simulink model "DinamicaActuadorTesis"  (R2021b)
settings: Solver=VariableStepAuto  StartTime=0.0  StopTime=5  RelTol=1e-3
libraries: slpidlib x4
(part 1 of 2)
settings Model: Creator=fabia  LastModifiedBy=fabia

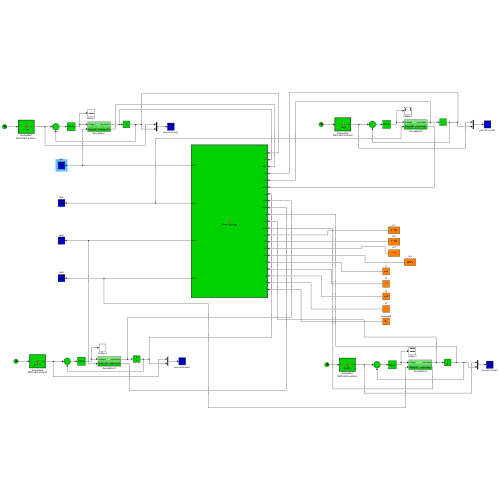
[thumbnail: Simulink's stored preview of the top-level diagram]
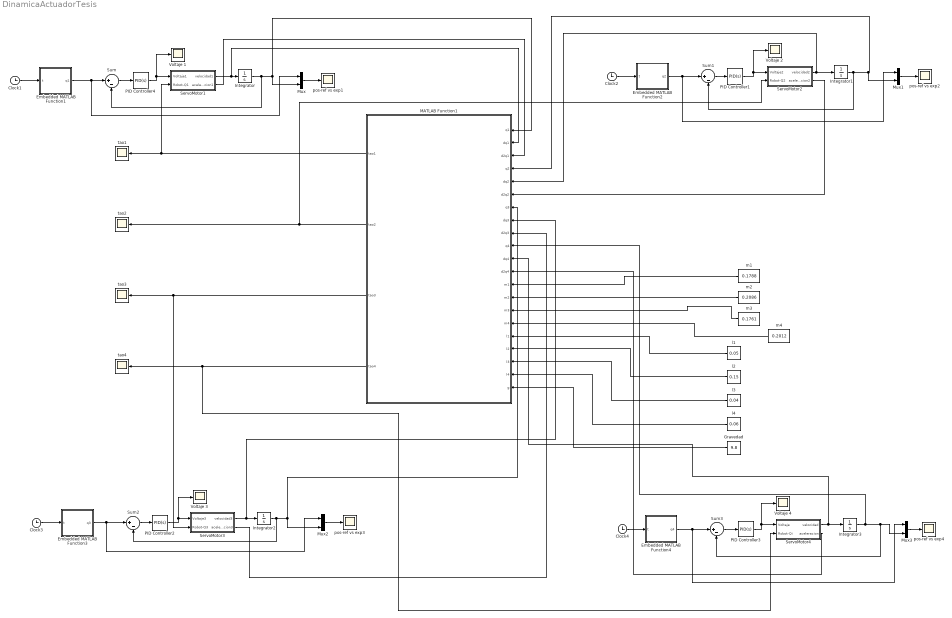
== system DinamicaActuadorTesis ==
  Clock{1..4} (4 alike) : Clock
      settings: Decimation=1000
  Embedded MATLAB Function1 : MATLAB Function  TreatAsAtomicUnit=on
  Embedded MATLAB Function2 : MATLAB Function  TreatAsAtomicUnit=on
  Embedded MATLAB Function3 : MATLAB Function  TreatAsAtomicUnit=on
  Embedded MATLAB Function4 : MATLAB Function  TreatAsAtomicUnit=on
  Gravedad : Constant  Value=9.8
  Integrator{,1..3} (4 alike) : Integrator
  MATLAB Function1 : MATLAB Function  TreatAsAtomicUnit=on
  Mux{,1..3} (4 alike) : Mux  Inputs=2
  PID Controller1 : slpidlib/PID Controller  Controller=PID  Form=Parallel  TimeDomain=Continuous-time  UseExternalTs=off  SampleTime=-1  IntegratorMethod=Forward Euler  FilterMethod=Forward Euler  ControllerParametersSource=internal  P=21468.8085757443  I=3151896.46029539  D=35.5661379721855  UseFilter=on  N=28467.1470128127  TunerSelectOption=Transfer Function Based (PID Tuner App)  InitialConditionSource=internal  InitialConditionForIntegrator=0  InitialConditionForFilter=0  DifferentiatorICPrevScaledInput=0  ExternalReset=none  TrackingMode=off  Kt=1  LimitOutput=off  SatLimitsSource=internal  UpperSaturationLimit=inf  LowerSaturationLimit=-inf  LinearizeAsGain=on  AntiWindupMode=none  Kb=1  POutMin=[]  POutMax=[]  IOutMin=[]  IOutMax=[]  DOutMin=[]  DOutMax=[]  NOutMin=[]  NOutMax=[]  SumOutMin=[]  SumOutMax=[]  SaturationOutMin=[]  SaturationOutMax=[]  PParamMin=[]  PParamMax=[]  IParamMin=[]  IParamMax=[]  DParamMin=[]  DParamMax=[]  NParamMin=[]  NParamMax=[]  KbParamMin=[]  KbParamMax=[]  KtParamMin=[]  KtParamMax=[]  KbOutMin=[]  KbOutMax=[]  KtOutMin=[]  KtOutMax=[]  IntegratorOutMin=[]  IntegratorOutMax=[]  FilterOutMin=[]  FilterOutMax=[]  SumI1OutMin=[]  SumI1OutMax=[]  SumI2OutMin=[]  SumI2OutMax=[]  SumI3OutMin=[]  SumI3OutMax=[]  SumI4OutMin=[]  SumI4OutMax=[]  SumDOutMin=[]  SumDOutMax=[]  DifferentiatorOutMin=[]  DifferentiatorOutMax=[]  FilterDiffOutCoefMin=[]  FilterDiffOutCoefMax=[]  ReciprocalOutMin=[]  ReciprocalOutMax=[]  SumDenOutMin=[]  SumDenOutMax=[]  SumNumOutMin=[]  SumNumOutMax=[]  DivideOutMin=[]  DivideOutMax=[]  UdiffTsProdOutMin=[]  UdiffTsProdOutMax=[]  NTsProdOutMin=[]  NTsProdOutMax=[]  UintegralTsProdOutMin=[]  UintegralTsProdOutMax=[]  UngainTsProdOutMin=[]  UngainTsProdOutMax=[]  IntegratorContinuousStateAttributes=''  IntegratorStateMustResolveToSignalObject=off  IntegratorRTWStateStorageClass=Auto  FilterContinuousStateAttributes=''  FilterStateMustResolveToSignalObject=off  FilterRTWStateStorageClass=Auto  ParallelPVariant=InternalParameters  IdealPVariant=Disabled  IVariant=InternalParameters  DVariant=InternalParameters  IntegratorVariant=Continuous  SatVariant=Disabled  AWVariant=Passthrough  PCopyVariant=Disabled  TRVariant=Disabled  FdbkBlocksVariant=Forward  IdealPFdbkVariant=Disabled  SatFdbkVariant=Disabled  DerivativeFilterVariant=ContFilter  NVariant=InternalParameters  NCopyVariant=Disabled  FilterICVariant=InternalICsFilter  IntegratorICVariant=InternalICs  ExternalResetVariant=Disabled  TRSumVariant=Passthrough  SumFdbkVariant=Disabled  SumVariant=Sum_PID  TsampFilterVariant=InternalTs  TsampNgainVariant=Passthrough  TsampIntegralVariant=Passthrough  ExternalSaturationOutDataTypeStr=Inherit: Same as second input
  PID Controller2 : slpidlib/PID Controller  Controller=PID  Form=Parallel  TimeDomain=Continuous-time  UseExternalTs=off  SampleTime=-1  IntegratorMethod=Forward Euler  FilterMethod=Forward Euler  ControllerParametersSource=internal  P=494.222408269061  I=42168.6852258058  D=0.963187955736722  UseFilter=on  N=2193.42887614857  TunerSelectOption=Transfer Function Based (PID Tuner App)  InitialConditionSource=internal  InitialConditionForIntegrator=0  InitialConditionForFilter=0  DifferentiatorICPrevScaledInput=0  ExternalReset=none  TrackingMode=off  Kt=1  LimitOutput=off  SatLimitsSource=internal  UpperSaturationLimit=inf  LowerSaturationLimit=-inf  LinearizeAsGain=on  AntiWindupMode=none  Kb=1  POutMin=[]  POutMax=[]  IOutMin=[]  IOutMax=[]  DOutMin=[]  DOutMax=[]  NOutMin=[]  NOutMax=[]  SumOutMin=[]  SumOutMax=[]  SaturationOutMin=[]  SaturationOutMax=[]  PParamMin=[]  PParamMax=[]  IParamMin=[]  IParamMax=[]  DParamMin=[]  DParamMax=[]  NParamMin=[]  NParamMax=[]  KbParamMin=[]  KbParamMax=[]  KtParamMin=[]  KtParamMax=[]  KbOutMin=[]  KbOutMax=[]  KtOutMin=[]  KtOutMax=[]  IntegratorOutMin=[]  IntegratorOutMax=[]  FilterOutMin=[]  FilterOutMax=[]  SumI1OutMin=[]  SumI1OutMax=[]  SumI2OutMin=[]  SumI2OutMax=[]  SumI3OutMin=[]  SumI3OutMax=[]  SumI4OutMin=[]  SumI4OutMax=[]  SumDOutMin=[]  SumDOutMax=[]  DifferentiatorOutMin=[]  DifferentiatorOutMax=[]  FilterDiffOutCoefMin=[]  FilterDiffOutCoefMax=[]  ReciprocalOutMin=[]  ReciprocalOutMax=[]  SumDenOutMin=[]  SumDenOutMax=[]  SumNumOutMin=[]  SumNumOutMax=[]  DivideOutMin=[]  DivideOutMax=[]  UdiffTsProdOutMin=[]  UdiffTsProdOutMax=[]  NTsProdOutMin=[]  NTsProdOutMax=[]  UintegralTsProdOutMin=[]  UintegralTsProdOutMax=[]  UngainTsProdOutMin=[]  UngainTsProdOutMax=[]  IntegratorContinuousStateAttributes=''  IntegratorStateMustResolveToSignalObject=off  IntegratorRTWStateStorageClass=Auto  FilterContinuousStateAttributes=''  FilterStateMustResolveToSignalObject=off  FilterRTWStateStorageClass=Auto  ParallelPVariant=InternalParameters  IdealPVariant=Disabled  IVariant=InternalParameters  DVariant=InternalParameters  IntegratorVariant=Continuous  SatVariant=Disabled  AWVariant=Passthrough  PCopyVariant=Disabled  TRVariant=Disabled  FdbkBlocksVariant=Forward  IdealPFdbkVariant=Disabled  SatFdbkVariant=Disabled  DerivativeFilterVariant=ContFilter  NVariant=InternalParameters  NCopyVariant=Disabled  FilterICVariant=InternalICsFilter  IntegratorICVariant=InternalICs  ExternalResetVariant=Disabled  TRSumVariant=Passthrough  SumFdbkVariant=Disabled  SumVariant=Sum_PID  TsampFilterVariant=InternalTs  TsampNgainVariant=Passthrough  TsampIntegralVariant=Passthrough  ExternalSaturationOutDataTypeStr=Inherit: Same as second input
  PID Controller3 : slpidlib/PID Controller  Controller=PID  Form=Parallel  TimeDomain=Continuous-time  UseExternalTs=off  SampleTime=-1  IntegratorMethod=Forward Euler  FilterMethod=Forward Euler  ControllerParametersSource=internal  P=494.222408269061  I=42168.6852258058  D=0.963187955736722  UseFilter=on  N=2193.42887614857  TunerSelectOption=Transfer Function Based (PID Tuner App)  InitialConditionSource=internal  InitialConditionForIntegrator=0  InitialConditionForFilter=0  DifferentiatorICPrevScaledInput=0  ExternalReset=none  TrackingMode=off  Kt=1  LimitOutput=off  SatLimitsSource=internal  UpperSaturationLimit=inf  LowerSaturationLimit=-inf  LinearizeAsGain=on  AntiWindupMode=none  Kb=1  POutMin=[]  POutMax=[]  IOutMin=[]  IOutMax=[]  DOutMin=[]  DOutMax=[]  NOutMin=[]  NOutMax=[]  SumOutMin=[]  SumOutMax=[]  SaturationOutMin=[]  SaturationOutMax=[]  PParamMin=[]  PParamMax=[]  IParamMin=[]  IParamMax=[]  DParamMin=[]  DParamMax=[]  NParamMin=[]  NParamMax=[]  KbParamMin=[]  KbParamMax=[]  KtParamMin=[]  KtParamMax=[]  KbOutMin=[]  KbOutMax=[]  KtOutMin=[]  KtOutMax=[]  IntegratorOutMin=[]  IntegratorOutMax=[]  FilterOutMin=[]  FilterOutMax=[]  SumI1OutMin=[]  SumI1OutMax=[]  SumI2OutMin=[]  SumI2OutMax=[]  SumI3OutMin=[]  SumI3OutMax=[]  SumI4OutMin=[]  SumI4OutMax=[]  SumDOutMin=[]  SumDOutMax=[]  DifferentiatorOutMin=[]  DifferentiatorOutMax=[]  FilterDiffOutCoefMin=[]  FilterDiffOutCoefMax=[]  ReciprocalOutMin=[]  ReciprocalOutMax=[]  SumDenOutMin=[]  SumDenOutMax=[]  SumNumOutMin=[]  SumNumOutMax=[]  DivideOutMin=[]  DivideOutMax=[]  UdiffTsProdOutMin=[]  UdiffTsProdOutMax=[]  NTsProdOutMin=[]  NTsProdOutMax=[]  UintegralTsProdOutMin=[]  UintegralTsProdOutMax=[]  UngainTsProdOutMin=[]  UngainTsProdOutMax=[]  IntegratorContinuousStateAttributes=''  IntegratorStateMustResolveToSignalObject=off  IntegratorRTWStateStorageClass=Auto  FilterContinuousStateAttributes=''  FilterStateMustResolveToSignalObject=off  FilterRTWStateStorageClass=Auto  ParallelPVariant=InternalParameters  IdealPVariant=Disabled  IVariant=InternalParameters  DVariant=InternalParameters  IntegratorVariant=Continuous  SatVariant=Disabled  AWVariant=Passthrough  PCopyVariant=Disabled  TRVariant=Disabled  FdbkBlocksVariant=Forward  IdealPFdbkVariant=Disabled  SatFdbkVariant=Disabled  DerivativeFilterVariant=ContFilter  NVariant=InternalParameters  NCopyVariant=Disabled  FilterICVariant=InternalICsFilter  IntegratorICVariant=InternalICs  ExternalResetVariant=Disabled  TRSumVariant=Passthrough  SumFdbkVariant=Disabled  SumVariant=Sum_PID  TsampFilterVariant=InternalTs  TsampNgainVariant=Passthrough  TsampIntegralVariant=Passthrough  ExternalSaturationOutDataTypeStr=Inherit: Same as second input
  PID Controller4 : slpidlib/PID Controller  Controller=PID  Form=Parallel  TimeDomain=Continuous-time  UseExternalTs=off  SampleTime=-1  IntegratorMethod=Forward Euler  FilterMethod=Forward Euler  ControllerParametersSource=internal  P=21468.8085757443  I=3151896.46029539  D=35.5661379721855  UseFilter=on  N=28467.1470128127  TunerSelectOption=Transfer Function Based (PID Tuner App)  InitialConditionSource=internal  InitialConditionForIntegrator=0  InitialConditionForFilter=0  DifferentiatorICPrevScaledInput=0  ExternalReset=none  TrackingMode=off  Kt=1  LimitOutput=off  SatLimitsSource=internal  UpperSaturationLimit=inf  LowerSaturationLimit=-inf  LinearizeAsGain=on  AntiWindupMode=none  Kb=1  POutMin=[]  POutMax=[]  IOutMin=[]  IOutMax=[]  DOutMin=[]  DOutMax=[]  NOutMin=[]  NOutMax=[]  SumOutMin=[]  SumOutMax=[]  SaturationOutMin=[]  SaturationOutMax=[]  PParamMin=[]  PParamMax=[]  IParamMin=[]  IParamMax=[]  DParamMin=[]  DParamMax=[]  NParamMin=[]  NParamMax=[]  KbParamMin=[]  KbParamMax=[]  KtParamMin=[]  KtParamMax=[]  KbOutMin=[]  KbOutMax=[]  KtOutMin=[]  KtOutMax=[]  IntegratorOutMin=[]  IntegratorOutMax=[]  FilterOutMin=[]  FilterOutMax=[]  SumI1OutMin=[]  SumI1OutMax=[]  SumI2OutMin=[]  SumI2OutMax=[]  SumI3OutMin=[]  SumI3OutMax=[]  SumI4OutMin=[]  SumI4OutMax=[]  SumDOutMin=[]  SumDOutMax=[]  DifferentiatorOutMin=[]  DifferentiatorOutMax=[]  FilterDiffOutCoefMin=[]  FilterDiffOutCoefMax=[]  ReciprocalOutMin=[]  ReciprocalOutMax=[]  SumDenOutMin=[]  SumDenOutMax=[]  SumNumOutMin=[]  SumNumOutMax=[]  DivideOutMin=[]  DivideOutMax=[]  UdiffTsProdOutMin=[]  UdiffTsProdOutMax=[]  NTsProdOutMin=[]  NTsProdOutMax=[]  UintegralTsProdOutMin=[]  UintegralTsProdOutMax=[]  UngainTsProdOutMin=[]  UngainTsProdOutMax=[]  IntegratorContinuousStateAttributes=''  IntegratorStateMustResolveToSignalObject=off  IntegratorRTWStateStorageClass=Auto  FilterContinuousStateAttributes=''  FilterStateMustResolveToSignalObject=off  FilterRTWStateStorageClass=Auto  ParallelPVariant=InternalParameters  IdealPVariant=Disabled  IVariant=InternalParameters  DVariant=InternalParameters  IntegratorVariant=Continuous  SatVariant=Disabled  AWVariant=Passthrough  PCopyVariant=Disabled  TRVariant=Disabled  FdbkBlocksVariant=Forward  IdealPFdbkVariant=Disabled  SatFdbkVariant=Disabled  DerivativeFilterVariant=ContFilter  NVariant=InternalParameters  NCopyVariant=Disabled  FilterICVariant=InternalICsFilter  IntegratorICVariant=InternalICs  ExternalResetVariant=Disabled  TRSumVariant=Passthrough  SumFdbkVariant=Disabled  SumVariant=Sum_PID  TsampFilterVariant=InternalTs  TsampNgainVariant=Passthrough  TsampIntegralVariant=Passthrough  ExternalSaturationOutDataTypeStr=Inherit: Same as second input
  ServoMotor1 : Subsystem
  ServoMotor2 : Subsystem
  ServoMotor3 : Subsystem
  ServoMotor4 : Subsystem
  Sum{,1..3} (4 alike) : Sum  Inputs=|+-
  Voltaje {1..4} (4 alike) : Scope
  l1 : Constant  Value=0.05
  l2 : Constant  Value=0.15
  l3 : Constant  Value=0.04
  l4 : Constant  Value=0.06
  m1 : Constant  Value=0.1788
  m2 : Constant  Value=0.2086
  m3 : Constant  Value=0.1761
  m4 : Constant  Value=0.2012
  pos-ref vs exp{1..4} (4 alike) : Scope
  tao{1..4} (4 alike) : Scope
  wires:
  Clock1/1 -> Embedded MATLAB Function1/1(t)
  Sum/1 -> PID Controller4/1
  Embedded MATLAB Function1/1(q1) -> Mux/1, Sum/1
  PID Controller4/1 -> Voltaje 1/1, ServoMotor1/1(Voltaje1)
  ServoMotor1/1(velocidad1) -> MATLAB Function1/2(dq1), Integrator/1
  Mux/1 -> pos-ref vs exp1/1
  Integrator/1 -> Mux/2, MATLAB Function1/1(q1), Sum/2
  l1/1 -> MATLAB Function1/17(l1)
  m1/1 -> MATLAB Function1/13(m1)
  ServoMotor1/2(aceleracion1) -> MATLAB Function1/3(d2q1)
  Mux1/1 -> pos-ref vs exp2/1
  PID Controller1/1 -> ServoMotor2/1(Voltaje2), Voltaje 2/1
  Clock2/1 -> Embedded MATLAB Function2/1(t)
  Embedded MATLAB Function2/1(q2) -> Mux1/1, Sum1/1
  ServoMotor2/1(velocidad2) -> MATLAB Function1/5(dq2), Integrator1/1
  Sum1/1 -> PID Controller1/1
  Integrator1/1 -> Mux1/2, MATLAB Function1/4(q2), Sum1/2
  Embedded MATLAB Function3/1(q3) -> Mux2/1, Sum2/1
  Sum2/1 -> PID Controller2/1
  Integrator2/1 -> Mux2/2, MATLAB Function1/7(q3), Sum2/2
  PID Controller2/1 -> ServoMotor3/1(Voltaje3), Voltaje 3/1
  Mux2/1 -> pos-ref vs exp3/1
  Clock3/1 -> Embedded MATLAB Function3/1(t)
  ServoMotor3/1(velocidad3) -> Integrator2/1, MATLAB Function1/8(dq3)
  ServoMotor4/1(velocidad) -> Integrator3/1, MATLAB Function1/11(dq4)
  Mux3/1 -> pos-ref vs exp4/1
  Sum3/1 -> PID Controller3/1
  Integrator3/1 -> MATLAB Function1/10(q4), Sum3/2, Mux3/2
  PID Controller3/1 -> ServoMotor4/1(Voltaje), Voltaje 4/1
  Embedded MATLAB Function4/1(q4) -> Mux3/1, Sum3/1
  MATLAB Function1/2(tao2) -> tao2/1, ServoMotor2/2(Robot-Q2)
  m2/1 -> MATLAB Function1/14(m2)
  l2/1 -> MATLAB Function1/18(l2)
  ServoMotor2/2(aceleracion2) -> MATLAB Function1/6(d2q2)
  MATLAB Function1/1(tao1) -> tao1/1, ServoMotor1/2(Robot-Q1)
  MATLAB Function1/3(tao3) -> tao3/1, ServoMotor3/2(Robot-Q3)
  MATLAB Function1/4(tao4) -> tao4/1, ServoMotor4/2(Robot-Qi)
  m3/1 -> MATLAB Function1/15(m3)
  l3/1 -> MATLAB Function1/19(l3)
  l4/1 -> MATLAB Function1/20(l4)
  Gravedad/1 -> MATLAB Function1/21(g)
  ServoMotor3/2(aceleracion3) -> MATLAB Function1/9(d2q3)
  m4/1 -> MATLAB Function1/16(m4)
  ServoMotor4/2(aceleracion) -> MATLAB Function1/12(d2q4)
  Clock4/1 -> Embedded MATLAB Function4/1(t)

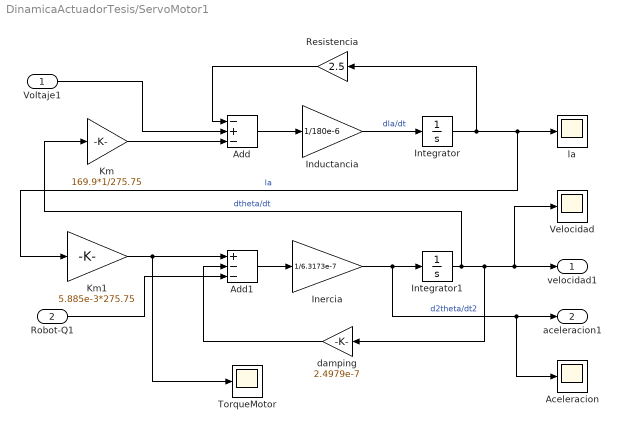
== system DinamicaActuadorTesis/ServoMotor1 ==
  Voltaje1 : Inport
  Robot-Q1 : Inport  Port=2
  Aceleracion : Scope
  Add : Sum  Inputs=-+-
  Add1 : Sum  Inputs=+--
  Inductancia : Gain  Gain=1/180e-6
  Inercia : Gain  Gain=1/6.3173e-7
  Integrator : Integrator
  Integrator1 : Integrator
  Km : Gain  Gain=169.9*1/275.75
  Km1 : Gain  Gain=5.885e-3*275.75
  Resistencia : Gain  Gain=2.5
  TorqueMotor : Scope
  Velocidad : Scope
  damping : Gain  Gain=2.4979e-7
  la : Scope
  velocidad1 : Outport
  aceleracion1 : Outport  Port=2
  wires:
  Voltaje1/1 -> Add/2
  Km/1 -> Add/3
  Resistencia/1 -> Add/1
  Add/1 -> Inductancia/1
  Inductancia/1 -> Integrator/1  "dla/dt"
  Integrator/1 -> Resistencia/1, la/1, Km1/1  "la"
  Add1/1 -> Inercia/1
  Inercia/1 -> Aceleracion/1, aceleracion1/1, Integrator1/1  "d2theta/dt2"
  Integrator1/1 -> Km/1, damping/1, Velocidad/1, velocidad1/1  "dtheta/dt"
  Robot-Q1/1 -> Add1/3
  damping/1 -> Add1/2
  Km1/1 -> TorqueMotor/1, Add1/1

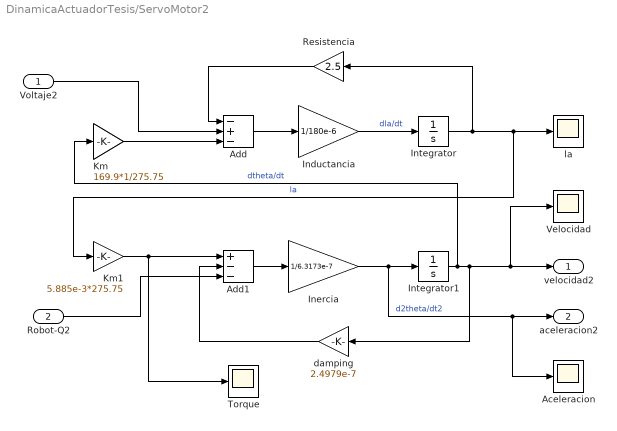
== system DinamicaActuadorTesis/ServoMotor2 ==
  Voltaje2 : Inport
  Robot-Q2 : Inport  Port=2
  Aceleracion : Scope
  Add : Sum  Inputs=-+-
  Add1 : Sum  Inputs=+--
  Inductancia : Gain  Gain=1/180e-6
  Inercia : Gain  Gain=1/6.3173e-7
  Integrator : Integrator
  Integrator1 : Integrator
  Km : Gain  Gain=169.9*1/275.75
  Km1 : Gain  Gain=5.885e-3*275.75
  Resistencia : Gain  Gain=2.5
  Torque : Scope
  Velocidad : Scope
  damping : Gain  Gain=2.4979e-7
  la : Scope
  velocidad2 : Outport
  aceleracion2 : Outport  Port=2
  wires:
  Voltaje2/1 -> Add/2
  Km/1 -> Add/3
  Resistencia/1 -> Add/1
  Add/1 -> Inductancia/1
  Inductancia/1 -> Integrator/1  "dla/dt"
  Integrator/1 -> Resistencia/1, la/1, Km1/1  "la"
  Add1/1 -> Inercia/1
  Inercia/1 -> Aceleracion/1, aceleracion2/1, Integrator1/1  "d2theta/dt2"
  Integrator1/1 -> Km/1, damping/1, Velocidad/1, velocidad2/1  "dtheta/dt"
  Robot-Q2/1 -> Add1/3
  damping/1 -> Add1/2
  Km1/1 -> Torque/1, Add1/1

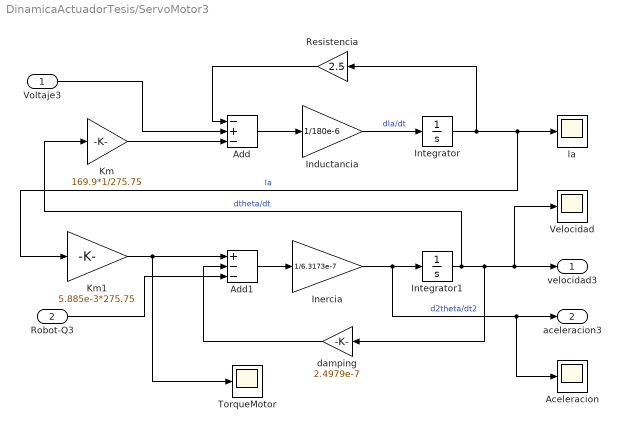
== system DinamicaActuadorTesis/ServoMotor3 ==
  Voltaje3 : Inport
  Robot-Q3 : Inport  Port=2
  Aceleracion : Scope
  Add : Sum  Inputs=-+-
  Add1 : Sum  Inputs=+--
  Inductancia : Gain  Gain=1/180e-6
  Inercia : Gain  Gain=1/6.3173e-7
  Integrator : Integrator
  Integrator1 : Integrator
  Km : Gain  Gain=169.9*1/275.75
  Km1 : Gain  Gain=5.885e-3*275.75
  Resistencia : Gain  Gain=2.5
  TorqueMotor : Scope
  Velocidad : Scope
  damping : Gain  Gain=2.4979e-7
  la : Scope
  velocidad3 : Outport
  aceleracion3 : Outport  Port=2
  wires:
  Voltaje3/1 -> Add/2
  Km/1 -> Add/3
  Resistencia/1 -> Add/1
  Add/1 -> Inductancia/1
  Inductancia/1 -> Integrator/1  "dla/dt"
  Integrator/1 -> Resistencia/1, la/1, Km1/1  "la"
  Add1/1 -> Inercia/1
  Inercia/1 -> Aceleracion/1, aceleracion3/1, Integrator1/1  "d2theta/dt2"
  Integrator1/1 -> Km/1, damping/1, Velocidad/1, velocidad3/1  "dtheta/dt"
  Robot-Q3/1 -> Add1/3
  damping/1 -> Add1/2
  Km1/1 -> TorqueMotor/1, Add1/1

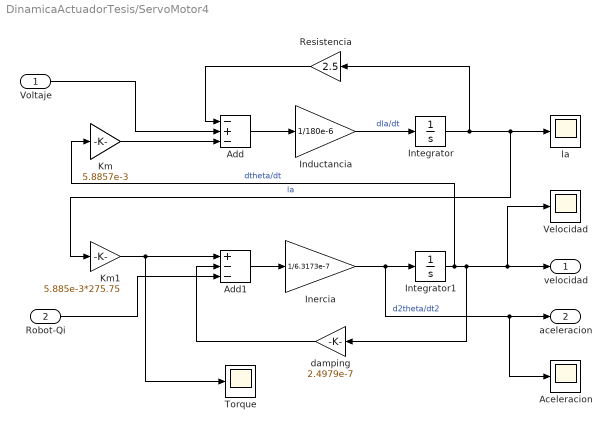
== system DinamicaActuadorTesis/ServoMotor4 ==
  Voltaje : Inport
  Robot-Qi : Inport  Port=2
  Aceleracion : Scope
  Add : Sum  Inputs=-+-
  Add1 : Sum  Inputs=+--
  Inductancia : Gain  Gain=1/180e-6
  Inercia : Gain  Gain=1/6.3173e-7
  Integrator : Integrator
  Integrator1 : Integrator
  Km : Gain  Gain=5.8857e-3
  Km1 : Gain  Gain=5.885e-3*275.75
  Resistencia : Gain  Gain=2.5
  Torque : Scope
  Velocidad : Scope
  damping : Gain  Gain=2.4979e-7
  la : Scope
  velocidad : Outport
  aceleracion : Outport  Port=2
  wires:
  Voltaje/1 -> Add/2
  Resistencia/1 -> Add/1
  Add1/1 -> Inercia/1
  Inductancia/1 -> Integrator/1  "dla/dt"
  Inercia/1 -> Aceleracion/1, aceleracion/1, Integrator1/1  "d2theta/dt2"
  Add/1 -> Inductancia/1
  Integrator/1 -> Resistencia/1, la/1, Km1/1  "la"
  Integrator1/1 -> Km/1, damping/1, Velocidad/1, velocidad/1  "dtheta/dt"
  Km1/1 -> Torque/1, Add1/1
  damping/1 -> Add1/2
  Km/1 -> Add/3
  Robot-Qi/1 -> Add1/3

== matlab function DinamicaActuadorTesis/Embedded MATLAB Function3 ==
  data: q3 output; t input
function q3 = posq3(t)
% This block supports an embeddable subset of the MATLAB language.
% See the help menu for details. 

if (t>=17)  % Si el t>=tmax, se repite una vez la rutina
    t=t-17;
end

if(t<6) % Movimiento 1
    t_inic = 0; % Tiempo en que inicia
    tf = 4;     % Tiempo en que termina
    y_ini = 1.570;
    y_f = -0.785;
elseif (t>=6 && t<12) % Movimiento 2
    t_inic = 6;
    tf = 4;
    y_ini = -0.785;
    y_f = -0.785;
else  % Movimiento 3
    t_inic = 12;
    tf = 5;
    y_ini = -0.785;
    y_f =  1.570;
end

% Calculo de trayectoria de tiempo minimo
Tb = tf/2;
% Vmax = 2*(y_f - y_ini)/(tf);
Vmax = (y_f - y_ini)/(tf - Tb);
ta = t - t_inic;
if(ta<0)
    q3 = y_ini;
elseif(ta >= 0 && ta < Tb)
    q3 = y_ini + (Vmax/(2*Tb))*ta*ta;
elseif(ta >= Tb && ta < (tf - Tb))
    q3 = (y_ini + y_f - Vmax*tf)/2 + Vmax*ta;
elseif(ta >= (tf - Tb) && ta < tf)
     q3 = y_f - (Vmax*(tf-ta)*(tf-ta)/(2*Tb));
else
    q3 = y_f;
end

== matlab function DinamicaActuadorTesis/Embedded MATLAB Function4 ==
  data: q4 output; t input
function q4 = posq4(t)
% This block supports an embeddable subset of the MATLAB language.
% See the help menu for details. 

if (t>=17)  % Si el t>=tmax, se repite una vez la rutina
    t=t-17;
end

if(t<6) % Movimiento 1
    t_inic = 0; % Tiempo en que inicia
    tf = 4;     % Tiempo en que termina
    y_ini = 1.570;
    y_f = -0.785;
elseif (t>=6 && t<12) % Movimiento 2
    t_inic = 6;
    tf = 4;
    y_ini = -0.785;
    y_f = -0.785;
else  % Movimiento 3
    t_inic = 12;
    tf = 5;
    y_ini = -0.785;
    y_f =  1.570;
end

% Calculo de trayectoria de tiempo minimo
Tb = tf/2;
% Vmax = 2*(y_f - y_ini)/(tf);
Vmax = (y_f - y_ini)/(tf - Tb);
ta = t - t_inic;
if(ta<0)
    q4 = y_ini;
elseif(ta >= 0 && ta < Tb)
    q4 = y_ini + (Vmax/(2*Tb))*ta*ta;
elseif(ta >= Tb && ta < (tf - Tb))
    q4 = (y_ini + y_f - Vmax*tf)/2 + Vmax*ta;
elseif(ta >= (tf - Tb) && ta < tf)
     q4 = y_f - (Vmax*(tf-ta)*(tf-ta)/(2*Tb));
else
    q4 = y_f;
end

== matlab function DinamicaActuadorTesis/Embedded MATLAB Function1 ==
  data: q1 output; t input
function q1 = posq1(t)
% This block supports an embeddable subset of the MATLAB language.
% See the help menu for details. 

if (t>=17)  % Si el t>=tmax, se repite otra vez la rutina
    t=t-17;
end

if(t<6) % Movimiento 1
    t_inic = 0; % Tiempo en que inicia
    tf = 4;     % Tiempo en que termina
    y_ini = 0;  % Posicion articular inicial (rad)
    y_f = -3.14159;    % Posicion articular final (rad)
elseif (t>=6 && t<12) % Movimiento 2
    t_inic = 6;
    tf = 4;
    y_ini = -3.14159;
    y_f =-3.14159;
else  % Movimiento 3
    t_inic = 12;
    tf = 5;
    y_ini =-3.14159;
    y_f = 0;
end

% Calculo de trayectoria de tiempo minimo
Tb = tf/2;  % el tb queda a la mitad del tiempo final

% Vmax = 2*(y_f - y_ini)/(tf);

Vmax = (y_f - y_ini)/(tf - Tb);
ta = t - t_inic;

% Polinomios que describen la curva en funcion de tiempo
if(ta<0)
    q1 = y_ini;
elseif(ta >= 0 && ta < Tb)
    q1 = y_ini + (Vmax/(2*Tb))*ta*ta;
elseif(ta >= Tb && ta < (tf - Tb))
    q1 = (y_ini + y_f - Vmax*tf)/2 + Vmax*ta;
elseif(ta >= (tf - Tb) && ta < tf)
     q1 = y_f - (Vmax*(tf-ta)*(tf-ta)/(2*Tb));
else
    q1 = y_f;
end

== matlab function DinamicaActuadorTesis/Embedded MATLAB Function2 ==
  data: q2 output; t input
function q2 = posq2(t)
% This block supports an embeddable subset of the MATLAB language.
% See the help menu for details. 

if (t>=17)  % Si el t>=tmax, se repite una vez la rutina
    t=t-17;
end

if(t<6) % Movimiento 1
    t_inic = 0; % Tiempo en que inicia
    tf = 4;     % Tiempo en que termina
    y_ini = 0.785;
    y_f = -1.570;
elseif (t>=6 && t<12) % Movimiento 2
    t_inic = 6;
    tf = 4;
    y_ini =  -1.5706;
    y_f =  -1.570;
else  % Movimiento 3
    t_inic = 12;
    tf = 5;
    y_ini =  -1.570;
    y_f = 0.785;
end

% Calculo de trayectoria de tiempo minimo
Tb = tf/2;
% Vmax = 2*(y_f - y_ini)/(tf);
Vmax = (y_f - y_ini)/(tf - Tb);
ta = t - t_inic;
if(ta<0)
    q2 = y_ini;
elseif(ta >= 0 && ta < Tb)
    q2 = y_ini + (Vmax/(2*Tb))*ta*ta;
elseif(ta >= Tb && ta < (tf - Tb))
    q2 = (y_ini + y_f - Vmax*tf)/2 + Vmax*ta;
elseif(ta >= (tf - Tb) && ta < tf)
     q2 = y_f - (Vmax*(tf-ta)*(tf-ta)/(2*Tb));
else
    q2 = y_f;
end
